simulink model "Power_split_controller_BC_Crane"  (R2021b)
settings: Solver=VariableStepAuto  StartTime=0.0  StopTime=262  RelTol=1
undefined symbols (not defined in the file): ISOC, ISOC_cr, P0, QC, QC_cr, R0, R0_cr, SOC_H, SOC_L, V0, V0_cr
libraries: ctrlSharedLib x1, simulink x1
settings Model: Creator=bldha  LastModifiedBy=bldha
settings SolverCC: ZeroCrossAlgorithm=Adaptive
settings DebuggingCC: IgnoredZcDiagnostic=none

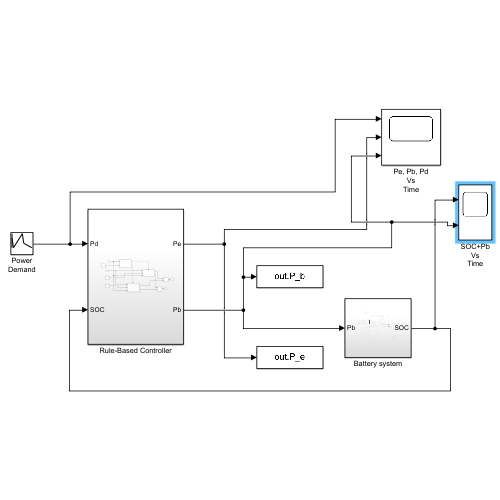
[thumbnail: Simulink's stored preview of the top-level diagram]
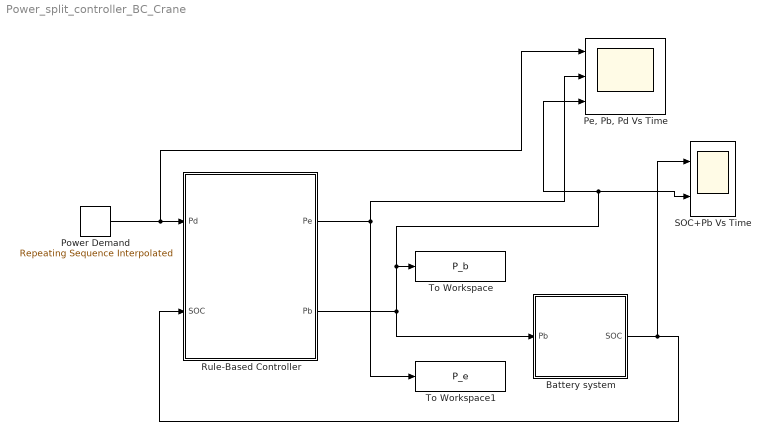
== system Power_split_controller_BC_Crane ==
  Battery system : Subsystem
  "Pe, Pb, Pd Vs Time" : Scope  NumInputPorts=3
  Power Demand : simulink/Sources/Repeating Sequence Interpolated  OutValues=Pd_cr.pow  TimeValues=Pd_cr.time  LookUpMeth=Interpolation-Use End Values  tsamp=1  OutMin=[]  OutMax=[]  OutDataTypeStr=double  OutputDataTypeScalingMode=double  OutDataType=fixdt(0,8)  OutScaling=2^-10
  Rule-Based Controller : Subsystem
  SOC+Pb Vs Time : Scope  NumInputPorts=2
  To Workspace : ToWorkspace  VariableName=P_b  SampleTime=-1
  To Workspace1 : ToWorkspace  VariableName=P_e  SampleTime=-1
  wires:
  Battery system/1(SOC) -> SOC+Pb Vs Time/1, Rule-Based Controller/2(SOC)
  Rule-Based Controller/1(Pe) -> To Workspace1/1, "Pe, Pb, Pd Vs Time"/2
  Power Demand/1 -> Rule-Based Controller/1(Pd), "Pe, Pb, Pd Vs Time"/1
  Rule-Based Controller/2(Pb) -> Battery system/1(Pb), To Workspace/1, SOC+Pb Vs Time/2, "Pe, Pb, Pd Vs Time"/3

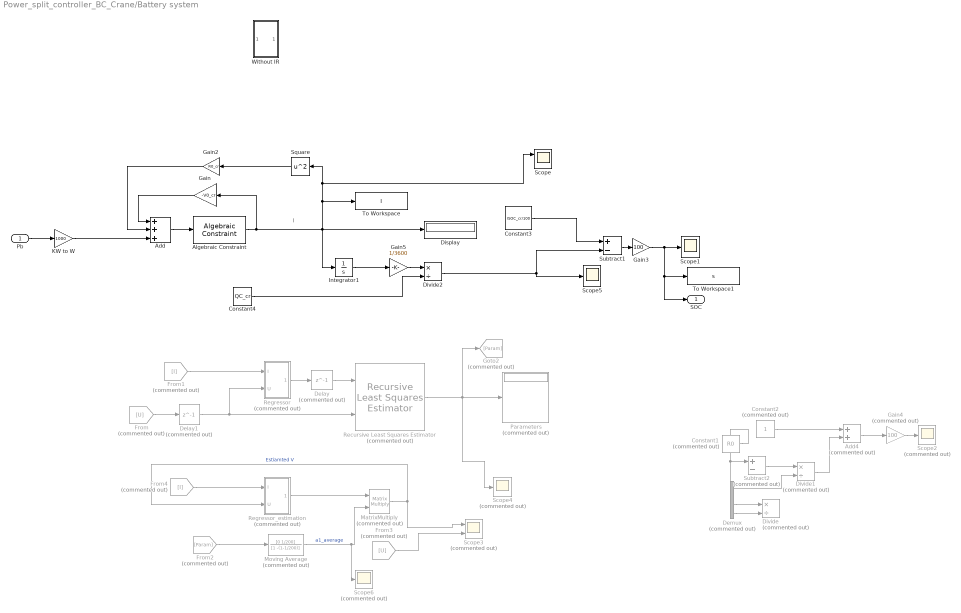
== system Power_split_controller_BC_Crane/Battery system ==
  note: I
  Pb : Inport
  Add : Sum  Inputs=+++
  Add4 : Sum  Commented=on
  Algebraic Constraint : AlgebraicConstraint  InitialGuess=-999999999999
  Constant1 : Constant  Commented=on  Value=R0
  Constant2 : Constant  Commented=on
  Constant3 : Constant  Value=ISOC_cr/100
  Constant4 : Constant  Value=QC_cr
  Delay : Delay  Commented=on  DelayLength=1  InitialCondition=1
  Delay1 : Delay  Commented=on  DelayLength=1  InitialCondition=1
  Demux : Demux  Commented=on
  Display : Display
  Divide : Product  Commented=on  Inputs=*/
  Divide1 : Product  Commented=on  Inputs=*/
  Divide2 : Product  Inputs=*/
  From : From  Commented=on  GotoTag=U
  From1 : From  Commented=on  GotoTag=I
  From2 : From  Commented=on  GotoTag=Param
  From3 : From  Commented=on  GotoTag=U
  From4 : From  Commented=on  GotoTag=I
  Gain : Gain  Gain=-V0_cr
  Gain2 : Gain  Gain=R0_cr
  Gain3 : Gain  Gain=100
  Gain4 : Gain  Commented=on  Gain=100
  Gain5 : Gain  Gain=1/3600
  Goto2 : Goto  Commented=on  GotoTag=Param
  Integrator1 : Integrator
  KW to W : Gain  Gain=1000
  MatrixMultiply : Product  Commented=on  Multiplication=Matrix(*)
  Moving Average : DiscreteFilter  Commented=on  Numerator=[0 1/200]  Denominator=[1 -(1-1/200)]
  Parameters : Display  Commented=on
  Recursive Least Squares Estimator : ctrlSharedLib/Recursive Least Squares Estimator  Commented=on  InitialEstimateSource=None  InitialParameterData=4  P0=2  InitialRegressors=0  InitialOutputs=0  History=Infinite  WindowLength=200  EstimationMethod=Forgetting Factor  AdaptationParameter=0.99  HasTimeVaryingAdaptationParameter=off  NormalizationBias=eps  OutputError=off  OutputP=off  AddEnablePort=off  InputProcessing=Sample-based  Ts=-1
      settings: SourceProductBaseCode=CT,ID
  Regressor : Subsystem  Commented=on
  Regressor_estimation : Subsystem  Commented=on
  Scope : Scope  NumInputPorts=2
  Scope1 : Scope
  Scope2 : Scope  Commented=on
  Scope3 : Scope  Commented=on  NumInputPorts=2
  Scope4 : Scope  Commented=on
  Scope5 : Scope
  Scope6 : Scope  Commented=on
  Square : Math  Operator=square  SaturateOnIntegerOverflow=on
  Subtract1 : Sum  Inputs=+-
  Subtract2 : Sum  Commented=on  Inputs=+-
  To Workspace : ToWorkspace  VariableName=I  SaveFormat=Structure With Time  SampleTime=-1
  To Workspace1 : ToWorkspace  VariableName=s  SaveFormat=Structure With Time  SampleTime=-1
  Without IR : Subsystem
  SOC : Outport
  wires:
  KW to W/1 -> Add/3
  Gain/1 -> Add/1
  Add/1 -> Algebraic Constraint/1
  Square/1 -> Gain2/1
  Gain2/1 -> Add/2
  Pb/1 -> KW to W/1
  Divide2/1 -> Subtract1/2, Scope5/1
  Constant3/1 -> Subtract1/1
  Subtract1/1 -> Gain3/1
  Gain3/1 -> To Workspace1/1, SOC/1, Scope1/1
  Constant4/1 -> Divide2/2
  Recursive Least Squares Estimator/1 -> Scope4/1, Goto2/1, Parameters/1
  From1/1 -> Regressor/1(I)
  Regressor/1(Out1) -> Delay/1
  Demux/3 -> Divide/1
  Demux/4 -> Divide/2
  Constant1/1 -> Divide1/2, Subtract2/1
  Subtract2/1 -> Divide1/1
  Constant2/1 -> Add4/1
  Divide1/1 -> Add4/2
  Add4/1 -> Gain4/1
  Gain4/1 -> Scope2/1
  Algebraic Constraint/1 -> Gain/1, Square/1, Scope/1, To Workspace/1, Display/1, Integrator1/1
  From4/1 -> Regressor_estimation/1(I)
  From2/1 -> Moving Average/1
  MatrixMultiply/1 -> Scope3/1, Regressor_estimation/2(U)  "Estiamted V"
  Regressor_estimation/1(Out1) -> MatrixMultiply/1
  Delay/1 -> Recursive Least Squares Estimator/1
  From/1 -> Delay1/1
  From3/1 -> Scope3/2
  Delay1/1 -> Regressor/2(U), Recursive Least Squares Estimator/2
  Moving Average/1 -> Scope6/1, MatrixMultiply/2  "a1_average"
  Gain5/1 -> Divide2/1
  Integrator1/1 -> Gain5/1

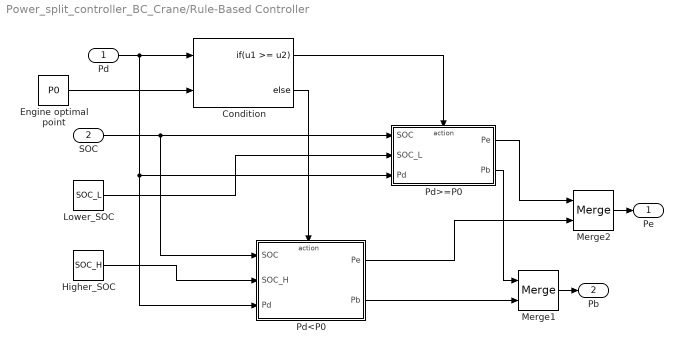
== system Power_split_controller_BC_Crane/Rule-Based Controller ==
  Pd : Inport
  SOC : Inport  Port=2
  "  Engine optimal point " : Constant  Value=P0
  Condition : If  NumInputs=2  IfExpression=u1 >= u2
  Higher_SOC : Constant  Value=SOC_H
  Lower_SOC : Constant  Value=SOC_L
  Merge1 : Merge
  Merge2 : Merge
  Pd<P0 : Subsystem  TreatAsAtomicUnit=on
  Pd>=P0 : Subsystem  TreatAsAtomicUnit=on
  Pe : Outport
  Pb : Outport  Port=2
  wires:
  SOC/1 -> Pd<P0/1(SOC), Pd>=P0/1(SOC)
  Merge1/1 -> Pb/1
  Pd/1 -> Condition/1, Pd<P0/3(Pd), Pd>=P0/3(Pd)
  "  Engine optimal point "/1 -> Condition/2
  Pd>=P0/2(Pb) -> Merge1/1
  Condition/2 -> Pd<P0/Action
  Lower_SOC/1 -> Pd>=P0/2(SOC_L)
  Condition/1 -> Pd>=P0/Action
  Higher_SOC/1 -> Pd<P0/2(SOC_H)
  Pd<P0/2(Pb) -> Merge1/2
  Merge2/1 -> Pe/1
  Pd>=P0/1(Pe) -> Merge2/1
  Pd<P0/1(Pe) -> Merge2/2

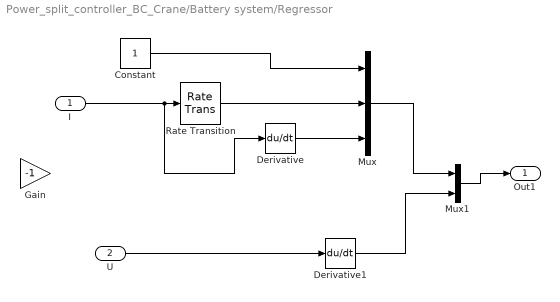
== system Power_split_controller_BC_Crane/Battery system/Regressor ==
  I : Inport
  U : Inport  Port=2
  Constant : Constant
  Derivative : Derivative
  Derivative1 : Derivative  CoefficientInTFapproximation=-inf
  Gain : Gain  Gain=-1
  Mux : Mux  Inputs=3
  Mux1 : Mux  Inputs=2
  Rate Transition : RateTransition  InitialCondition=1
  Out1 : Outport
  wires:
  Mux1/1 -> Out1/1
  Mux/1 -> Mux1/1
  Constant/1 -> Mux/1
  Derivative/1 -> Mux/3
  Derivative1/1 -> Mux1/2
  U/1 -> Derivative1/1
  I/1 -> Derivative/1, Rate Transition/1
  Rate Transition/1 -> Mux/2

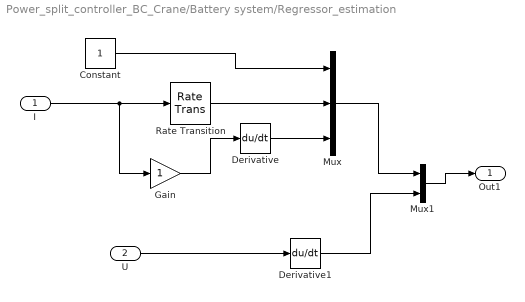
== system Power_split_controller_BC_Crane/Battery system/Regressor_estimation ==
  I : Inport
  U : Inport  Port=2
  Constant : Constant
  Derivative : Derivative
  Derivative1 : Derivative  CoefficientInTFapproximation=-inf
  Gain : Gain
  Mux : Mux  Inputs=3
  Mux1 : Mux  Inputs=2
  Rate Transition : RateTransition
  Out1 : Outport
  wires:
  I/1 -> Gain/1, Rate Transition/1
  U/1 -> Derivative1/1
  Derivative1/1 -> Mux1/2
  Derivative/1 -> Mux/3
  Constant/1 -> Mux/1
  Mux/1 -> Mux1/1
  Mux1/1 -> Out1/1
  Rate Transition/1 -> Mux/2
  Gain/1 -> Derivative/1

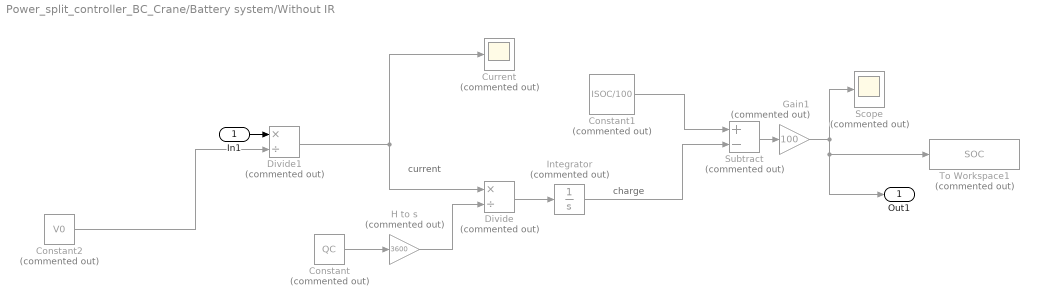
== system Power_split_controller_BC_Crane/Battery system/Without IR ==
  note: current
  note: charge
  In1 : Inport
  Constant : Constant  Commented=on  Value=QC
  Constant1 : Constant  Commented=on  Value=ISOC/100
  Constant2 : Constant  Commented=on  Value=V0
  Current : Scope  Commented=on
  Divide : Product  Commented=on  Inputs=*/
  Divide1 : Product  Commented=on  Inputs=*/
  Gain1 : Gain  Commented=on  Gain=100
  H to s : Gain  Commented=on  Gain=3600
  Integrator : Integrator  Commented=on
  Scope : Scope  Commented=on
  Subtract : Sum  Commented=on  Inputs=+-
  To Workspace1 : ToWorkspace  Commented=on  VariableName=SOC  SampleTime=-1
  Out1 : Outport
  wires:
  Subtract/1 -> Gain1/1
  Constant2/1 -> Divide1/2
  Gain1/1 -> Out1/1, To Workspace1/1, Scope/1
  Constant/1 -> H to s/1
  Divide1/1 -> Divide/1, Current/1
  H to s/1 -> Divide/2
  Divide/1 -> Integrator/1
  Integrator/1 -> Subtract/2
  Constant1/1 -> Subtract/1
  In1/1 -> Divide1/1

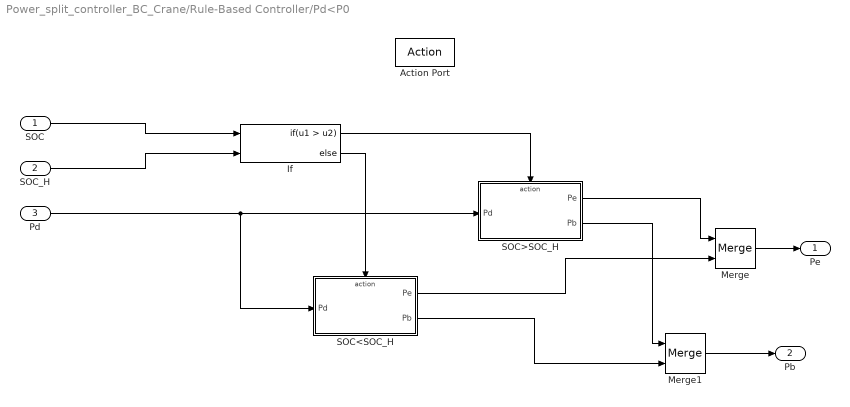
== system Power_split_controller_BC_Crane/Rule-Based Controller/Pd<P0 ==
  SOC : Inport
  SOC_H : Inport  Port=2
  Pd : Inport  Port=3
  Action Port : ActionPort  ActionPortLabel=else
  If : If  NumInputs=2  IfExpression=u1 > u2
  Merge : Merge
  Merge1 : Merge
  SOC<SOC_H : Subsystem  TreatAsAtomicUnit=on
  SOC>SOC_H : Subsystem  TreatAsAtomicUnit=on
  Pe : Outport
  Pb : Outport  Port=2
  wires:
  Pd/1 -> SOC<SOC_H/1(Pd), SOC>SOC_H/1(Pd)
  SOC>SOC_H/2(Pb) -> Merge1/1
  SOC_H/1 -> If/2
  SOC/1 -> If/1
  Merge1/1 -> Pb/1
  If/1 -> SOC>SOC_H/Action
  SOC>SOC_H/1(Pe) -> Merge/1
  SOC<SOC_H/1(Pe) -> Merge/2
  SOC<SOC_H/2(Pb) -> Merge1/2
  If/2 -> SOC<SOC_H/Action
  Merge/1 -> Pe/1

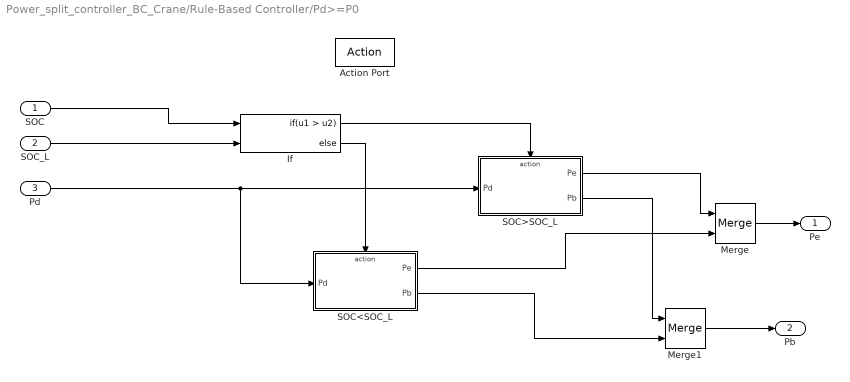
== system Power_split_controller_BC_Crane/Rule-Based Controller/Pd>=P0 ==
  SOC : Inport
  SOC_L : Inport  Port=2
  Pd : Inport  Port=3
  Action Port : ActionPort  ActionPortLabel=if(u1 >= u2)
  If : If  NumInputs=2  IfExpression=u1 > u2
  Merge : Merge
  Merge1 : Merge
  SOC<SOC_L : Subsystem  TreatAsAtomicUnit=on
  SOC>SOC_L : Subsystem  TreatAsAtomicUnit=on
  Pe : Outport
  Pb : Outport  Port=2
  wires:
  SOC/1 -> If/1
  SOC_L/1 -> If/2
  If/1 -> SOC>SOC_L/Action
  If/2 -> SOC<SOC_L/Action
  SOC>SOC_L/1(Pe) -> Merge/1
  SOC<SOC_L/1(Pe) -> Merge/2
  Merge/1 -> Pe/1
  SOC>SOC_L/2(Pb) -> Merge1/1
  SOC<SOC_L/2(Pb) -> Merge1/2
  Merge1/1 -> Pb/1
  Pd/1 -> SOC<SOC_L/1(Pd), SOC>SOC_L/1(Pd)

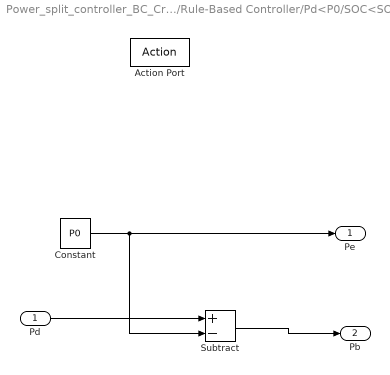
== system Power_split_controller_BC_Crane/Rule-Based Controller/Pd<P0/SOC<SOC_H ==
  Pd : Inport
  Action Port : ActionPort  ActionPortLabel=else
  Constant : Constant  Value=P0
  Subtract : Sum  Inputs=+-
  Pe : Outport
  Pb : Outport  Port=2
  wires:
  Subtract/1 -> Pb/1
  Pd/1 -> Subtract/1
  Constant/1 -> Subtract/2, Pe/1

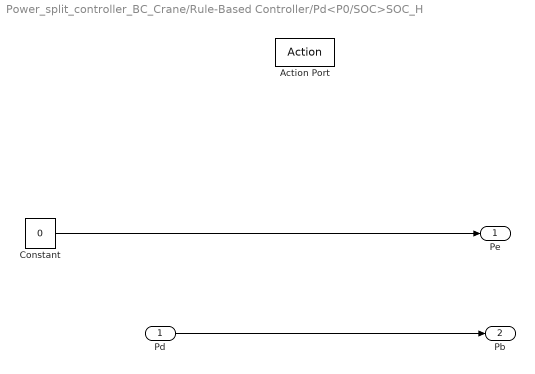
== system Power_split_controller_BC_Crane/Rule-Based Controller/Pd<P0/SOC>SOC_H ==
  Pd : Inport
  Action Port : ActionPort  ActionPortLabel=if(u1 > u2)
  Constant : Constant  Value=0
  Pe : Outport
  Pb : Outport  Port=2
  wires:
  Constant/1 -> Pe/1
  Pd/1 -> Pb/1

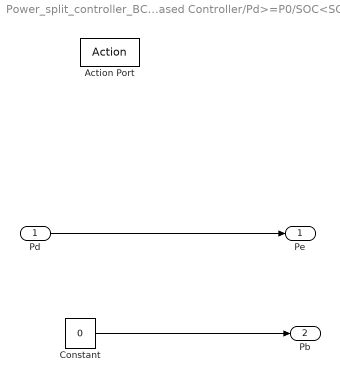
== system Power_split_controller_BC_Crane/Rule-Based Controller/Pd>=P0/SOC<SOC_L ==
  Pd : Inport
  Action Port : ActionPort  ActionPortLabel=else
  Constant : Constant  Value=0
  Pe : Outport
  Pb : Outport  Port=2
  wires:
  Constant/1 -> Pb/1
  Pd/1 -> Pe/1

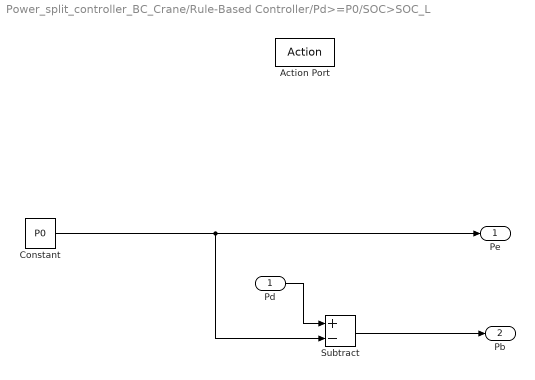
== system Power_split_controller_BC_Crane/Rule-Based Controller/Pd>=P0/SOC>SOC_L ==
  Pd : Inport
  Action Port : ActionPort  ActionPortLabel=if(u1 > u2)
  Constant : Constant  Value=P0
  Subtract : Sum  Inputs=+-
  Pe : Outport
  Pb : Outport  Port=2
  wires:
  Constant/1 -> Subtract/2, Pe/1
  Pd/1 -> Subtract/1
  Subtract/1 -> Pb/1
